simulink model "LLC_FullBridge"  (R2020b)
settings: Solver=VariableStepAuto  StartTime=0.0  StopTime=0.005  MaxStep=1e-4  RelTol=1e-4  EnableMultiTasking=on
PreLoadFcn:
  | Ts_Control=25e-6;
  | Rs_fet=1e8;  % FET snubber resistance (ohms)
  | Cs_fet=inf;  % FET snubber capacitance (ohms)
  | Vf=0.6;        % Diode forward voltage (V)
InitFcn:
  | Ts_Control=25e-6;
libraries: powerlib x24, powerlib_meascontrol x3, pid_lib x1
Description:
  | Copyright 2008-2019 The MathWorks, Inc.
settings Model: SimulationMode=accelerator  Creator=MathWorks  LastModifiedBy=lauramarks2
settings SolverCC: SolverResetMethod=Robust
settings DataIOCC: ReturnWorkspaceOutputs=off
settings OptimizationCC: LifeSpan=inf
settings DebuggingCC: SFUnexpectedBacktrackingDiag=warning  SFNoUnconditionalDefaultTransitionDiag=warning  SFExecutionAtInitializationDiag=none  ArithmeticOperatorsInVariantConditions=warning
settings SFSimCC: SimUseLocalCustomCode=off  CustomCodeUndefinedFunction=UseInterfaceOnly
settings RTWCC: RTWUseLocalCustomCode=off
settings CodeAppCC: StateflowObjectComments=on
settings GRTTargetCC: TargetLangStandard=C89/C90 (ANSI)
settings ConfigComp: CovMetricSettings=dw  CovSaveCumulativeToWorkspaceVar=on  CovSaveSingleToWorkspaceVar=on  CovExternalEMLEnable=off
settings SimscapeCC: SimscapeNormalizeSystem=off  SimscapeNominalValues={1, 'bar'; 1, 'cm^3/s'; 1, 'bar*kg/s'; 1, 'kJ/kg'; 1, 'kW'; }

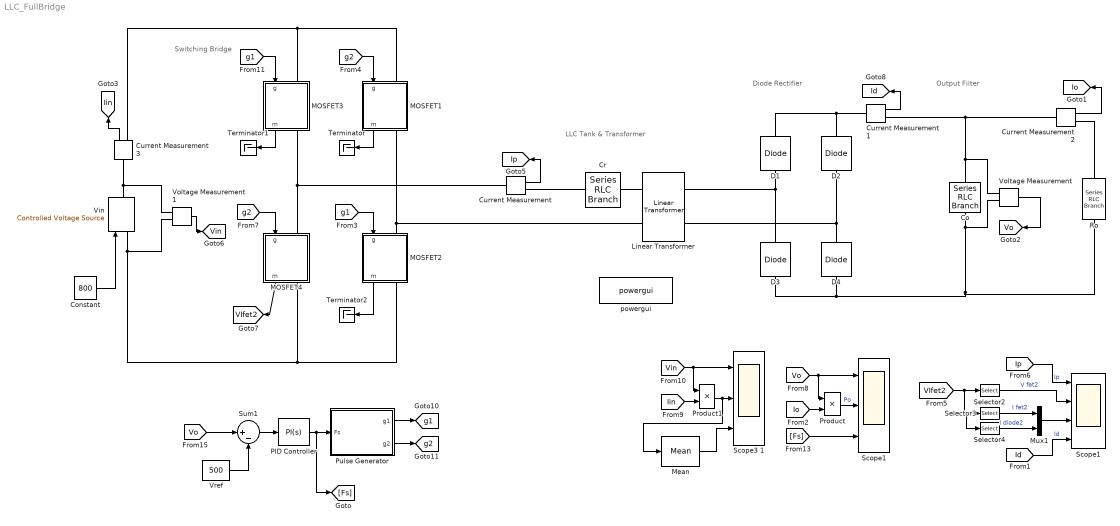
== system LLC_FullBridge ==
  note: LLC Tank & Transformer
  note: Diode
      | Rectifier
  note: Switching
      | Bridge
  note: Output
      | Filter
  Co : powerlib/Elements/Series RLC Branch  LConnTagsString=__new0  RConnTagsString=__new0  BranchType=C  Resistance=1e-4  Inductance=200e-6  SetiL0=off  InitialCurrent=0  Capacitance=100e-6  Setx0=on  InitialVoltage=24  Measurements=None
  Constant : Constant  Value=800  OutDataTypeStr=double
  Cr : powerlib/Elements/Series RLC Branch  LConnTagsString=__new0  RConnTagsString=__new0  BranchType=C  Resistance=1e-4  Inductance=200e-6  SetiL0=off  InitialCurrent=0  Capacitance=1.5e-6  Setx0=off  InitialVoltage=40  Measurements=None
  Current Measurement{,1..3} (4 alike) : powerlib/Measurements/Current Measurement  PhasorSimulation=off  OutputType=Complex  PSBequivalent=0
  D{1..4} (4 alike) : powerlib/Power Electronics/Diode  Ron=1e-3  Lon=0  Vf=0.5  IC=0  UseSnubber=off  Rs=1e6  Cs=inf  Measurements=off
  Linear Transformer : powerlib/Elements/Linear Transformer  UNITS=SI  NominalPower=[ 100e3 85e3 ]  winding1="[8   1e-2  2.02e-6]"  winding2="[6  1e-2  1.16e-6 ]"  ThreeWindings=off  winding3=[3.15e+05 0.7938 0.084225]  RmLm=[1e4 963e-6]  Measurements=None  DataType=on
  MOSFET1 : Subsystem
  MOSFET2 : Subsystem
  MOSFET3 : Subsystem
  MOSFET4 : Subsystem
  Mean : powerlib_meascontrol/Measurements/Mean  Freq=89.2e3  Vinit=0  Ts=0
  Mux1 : Mux  Inputs=2
  PID Controller : pid_lib/PID Controller  Controller=PI  Form=Parallel  TimeDomain=Continuous-time  UseExternalTs=off  SampleTime=-1  IntegratorMethod=Forward Euler  FilterMethod=Forward Euler  ControllerParametersSource=internal  P=1300  I=1e-3  D=0  UseFilter=on  N=100  TunerSelectOption=Transfer Function Based (PID Tuner App)  InitialConditionSource=internal  InitialConditionForIntegrator=89e3  InitialConditionForFilter=0  DifferentiatorICPrevScaledInput=0  ExternalReset=none  TrackingMode=off  Kt=1  LimitOutput=off  SatLimitsSource=internal  UpperSaturationLimit=inf  LowerSaturationLimit=0  LinearizeAsGain=on  AntiWindupMode=none  Kb=1  POutMin=[]  POutMax=[]  IOutMin=[]  IOutMax=[]  DOutMin=[]  DOutMax=[]  NOutMin=[]  NOutMax=[]  SumOutMin=[]  SumOutMax=[]  SaturationOutMin=[]  SaturationOutMax=[]  PParamMin=[]  PParamMax=[]  IParamMin=[]  IParamMax=[]  DParamMin=[]  DParamMax=[]  NParamMin=[]  NParamMax=[]  KbParamMin=[]  KbParamMax=[]  KtParamMin=[]  KtParamMax=[]  KbOutMin=[]  KbOutMax=[]  KtOutMin=[]  KtOutMax=[]  IntegratorOutMin=[]  IntegratorOutMax=[]  FilterOutMin=[]  FilterOutMax=[]  SumI1OutMin=[]  SumI1OutMax=[]  SumI2OutMin=[]  SumI2OutMax=[]  SumI3OutMin=[]  SumI3OutMax=[]  SumI4OutMin=[]  SumI4OutMax=[]  SumDOutMin=[]  SumDOutMax=[]  DifferentiatorOutMin=[]  DifferentiatorOutMax=[]  FilterDiffOutCoefMin=[]  FilterDiffOutCoefMax=[]  ReciprocalOutMin=[]  ReciprocalOutMax=[]  SumDenOutMin=[]  SumDenOutMax=[]  SumNumOutMin=[]  SumNumOutMax=[]  DivideOutMin=[]  DivideOutMax=[]  UdiffTsProdOutMin=[]  UdiffTsProdOutMax=[]  NTsProdOutMin=[]  NTsProdOutMax=[]  UintegralTsProdOutMin=[]  UintegralTsProdOutMax=[]  UngainTsProdOutMin=[]  UngainTsProdOutMax=[]  IntegratorContinuousStateAttributes=''  IntegratorStateMustResolveToSignalObject=off  IntegratorRTWStateStorageClass=Auto  FilterContinuousStateAttributes=''  FilterStateMustResolveToSignalObject=off  FilterRTWStateStorageClass=Auto  ParallelPVariant=InternalParameters  IdealPVariant=Disabled  IVariant=InternalParameters  DVariant=Disabled  IntegratorVariant=Continuous  SatVariant=Disabled  AWVariant=Passthrough  PCopyVariant=Disabled  TRVariant=Disabled  FdbkBlocksVariant=Forward  IdealPFdbkVariant=Disabled  SatFdbkVariant=Disabled  DerivativeFilterVariant=Disabled  NVariant=Disabled  NCopyVariant=Disabled_SignalSpec  FilterICVariant=Disabled  IntegratorICVariant=InternalICs  ExternalResetVariant=Disabled  TRSumVariant=Passthrough  SumFdbkVariant=Disabled  SumVariant=Sum_PI  TsampFilterVariant=InternalTs  TsampNgainVariant=Passthrough  TsampIntegralVariant=Passthrough  ExternalSaturationOutDataTypeStr=Inherit: Same as second input
  Product : Product
  Product1 : Product
  Pulse Generator : Subsystem
  Ro : powerlib/Elements/Series RLC Branch  LConnTagsString=__new0  RConnTagsString=__new0  BranchType=R  Resistance=2.5  Inductance=200e-6  SetiL0=off  InitialCurrent=0  Capacitance=400e-6  Setx0=off  InitialVoltage=0  Measurements=Branch voltage and current
  Scope1 : Scope  NumInputPorts=4
  "Scope1 " : Scope  NumInputPorts=3
  Scope3 1 : Scope  NumInputPorts=3
  Selector2 : Selector  InputPortWidth=3  IndexOptions=Index vector (dialog)  Indices=2  OutputSizes=1
  Selector3 : Selector  InputPortWidth=3  IndexOptions=Index vector (dialog)  Indices=1  OutputSizes=1
  Selector4 : Selector  InputPortWidth=3  IndexOptions=Index vector (dialog)  Indices=3  OutputSizes=1
  Sum1 : Sum  Inputs=|+-  InputSameDT=on  SaturateOnIntegerOverflow=on  OutDataTypeStr=Inherit: Same as first input
  Terminator : Terminator
  Terminator1 : Terminator
  Terminator2 : Terminator
  "Vin " : powerlib/Electrical Sources/Controlled Voltage Source  Initialize=on  Source_Type=AC  Amplitude=0  Phase=0  Frequency=0  Measurements=None
  Voltage Measurement : powerlib/Measurements/Voltage Measurement  PhasorSimulation=off  OutputType=Complex  PSBequivalent=0
  Voltage Measurement1 : powerlib/Measurements/Voltage Measurement  PhasorSimulation=off  OutputType=Complex  PSBequivalent=0
  Vref : Constant  Value=500
  powergui : powerlib/powergui  Priority=1  SimulationMode=Continuous  SampleTime=5e-9  frequency=60  Iterations=50  frequencyindice=0  Pbase=100e6  ErrMax=1e-4  UnitsV=kV  UnitsW=MW  buscounter=0  FunctionMessages=on  echomessages=off  EnableUseOfTLC=off  CurrentSourceSwitches=off  DisableSnubberDevices=off  DisableRonSwitches=off  DisableVfSwitches=off  DisplayEquations=off  AutomaticDiscreteSolvers=off  SolverType=Tustin/Backward Euler (TBE)  Interpol=off  ExternalGateDelay=off  methode=off  Ts=100  x0status=blocks  SPID=on  SwTol=0  HookPort=off  NonlinearTolerance=0  nMaxIteration=15  ContinueOnMaxIteration=off  RestoreLinks=warning  ResistiveCurrentMeasurement=off  Frange=[0:2:500]  Ylog=off  Xlog=on  ShowGrid=off  save=off  variable=ZData  structure=0  ZoomFFT=off  StartTime=0.0  cycles=1  DisplayStyle=1  fundamental=60  FreqAxis=off  MaxFrequency=1000  frequencyindicesteady=1  RmsSteady=1  display=off
  tag scope: Id=global, Iin=global, Io=global, Ip=global, VIfet2=global, Vin=global, Vo=global, g1=global, g2=global
  wires:
  [g1] -> MOSFET2/1(g)
  [g2] -> MOSFET1/1(g)
  Current Measurement/1 -> [Ip]
  Voltage Measurement/1 -> [Vo]
  Current Measurement1/1 -> [Id]
  [Vo] -> Product/1, "Scope1 "/1
  Pulse Generator/1(g1) -> [g1]
  Pulse Generator/2(g2) -> [g2]
  [Fs] -> "Scope1 "/3
  MOSFET1/1(m) -> Terminator/1
  [VIfet2] -> Selector4/1, Selector3/1, Selector2/1
  Mux1/1 -> Scope1/3
  Selector4/1 -> Mux1/2  "I diode2"
  Selector3/1 -> Mux1/1  "I fet2"
  [Id] -> Scope1/4  "Id"
  Selector2/1 -> Scope1/2  "V fet2"
  [Ip] -> Scope1/1  "Ip"
  Current Measurement2/1 -> [Io]
  Product/1 -> "Scope1 "/2  "Po"
  [Io] -> Product/2
  [Vo] -> Sum1/1
  Vref/1 -> Sum1/2
  PID Controller/1 -> [Fs], Pulse Generator/1(Fs)
  Constant/1 -> "Vin "/1
  Sum1/1 -> PID Controller/1
  Current Measurement3/1 -> [Iin]
  [Vin] -> Product1/1, Scope3 1/1
  [Iin] -> Product1/2
  Product1/1 -> Mean/1, Scope3 1/2
  Voltage Measurement1/1 -> [Vin]
  Mean/1 -> Scope3 1/3
  [g2] -> MOSFET4/1(g)
  MOSFET4/1(m) -> [VIfet2]
  [g1] -> MOSFET3/1(g)
  MOSFET3/1(m) -> Terminator1/1
  MOSFET2/1(m) -> Terminator2/1
  connections:
  Co/RConn1 -- Voltage Measurement/LConn2 -- Ro/RConn1 -- D4/LConn1 -- D3/LConn1
  Linear Transformer/RConn1 -- D3/RConn1 -- D1/LConn1
  MOSFET2/LConn1 -- Linear Transformer/LConn2 -- MOSFET1/RConn1
  Linear Transformer/RConn2 -- D4/RConn1 -- D2/LConn1
  MOSFET1/LConn1 -- MOSFET3/LConn1 -- Current Measurement3/RConn1
  "Vin "/LConn1 -- Voltage Measurement1/LConn2 -- MOSFET2/RConn1 -- MOSFET4/RConn1
  Cr/LConn1 -- Current Measurement/RConn1
  Linear Transformer/LConn1 -- Cr/RConn1
  D1/RConn1 -- D2/RConn1 -- Current Measurement1/LConn1
  Voltage Measurement/LConn1 -- Current Measurement2/LConn1 -- Current Measurement1/RConn1 -- Co/LConn1
  Current Measurement2/RConn1 -- Ro/LConn1
  Current Measurement3/LConn1 -- Voltage Measurement1/LConn1 -- "Vin "/RConn1
  MOSFET4/LConn1 -- Current Measurement/LConn1 -- MOSFET3/RConn1

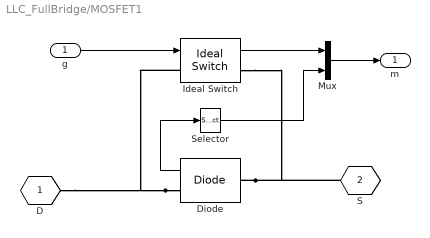
== system LLC_FullBridge/MOSFET1 ==
  g : Inport
  Diode : powerlib/Power Electronics/Diode  Ron=1e-3  Lon=0  Vf=Vf  IC=0  UseSnubber=0  Rs=inf  Cs=0  Measurements=on
  Ideal Switch : powerlib/Power Electronics/Ideal Switch  Ron=1e-3  Lon=0  IC=0  Rs=Rs_fet  Cs=Cs_fet  Measurements=on
  Mux : Mux  Inputs=[2,1]
  Selector : Selector  InputPortWidth=2  IndexOptions=Index vector (dialog)  Indices=1  OutputSizes=1
  D : PMIOPort  Tag=PMCPort  Side=Left
  S : PMIOPort  Tag=PMCPort  Port=2  Side=Right
  m : Outport  VectorParamsAs1DForOutWhenUnconnected=off
  wires:
  Diode/1 -> Selector/1
  g/1 -> Ideal Switch/1
  Ideal Switch/1 -> Mux/1
  Selector/1 -> Mux/2
  Mux/1 -> m/1
  connections:
  Diode/LConn1 -- S/RConn1 -- Ideal Switch/RConn1
  Diode/RConn1 -- D/RConn1 -- Ideal Switch/LConn1

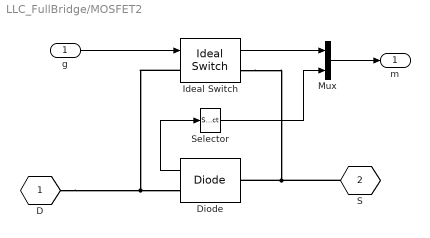
== system LLC_FullBridge/MOSFET2 ==
  g : Inport
  Diode : powerlib/Power Electronics/Diode  Ron=1e-3  Lon=0  Vf=Vf  IC=0  UseSnubber=0  Rs=inf  Cs=0  Measurements=on
  Ideal Switch : powerlib/Power Electronics/Ideal Switch  Ron=1e-3  Lon=0  IC=0  Rs=Rs_fet  Cs=Cs_fet  Measurements=on
  Mux : Mux  Inputs=[2,1]
  Selector : Selector  InputPortWidth=2  IndexOptions=Index vector (dialog)  Indices=1  OutputSizes=1
  D : PMIOPort  Tag=PMCPort  Side=Left
  S : PMIOPort  Tag=PMCPort  Port=2  Side=Right
  m : Outport  VectorParamsAs1DForOutWhenUnconnected=off
  wires:
  Mux/1 -> m/1
  Selector/1 -> Mux/2
  Ideal Switch/1 -> Mux/1
  g/1 -> Ideal Switch/1
  Diode/1 -> Selector/1
  connections:
  Ideal Switch/LConn1 -- D/RConn1 -- Diode/RConn1
  Ideal Switch/RConn1 -- S/RConn1 -- Diode/LConn1

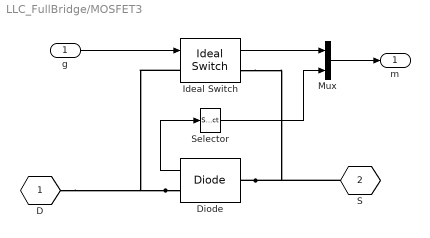
== system LLC_FullBridge/MOSFET3 ==
  g : Inport
  Diode : powerlib/Power Electronics/Diode  Ron=1e-3  Lon=0  Vf=Vf  IC=0  UseSnubber=0  Rs=inf  Cs=0  Measurements=on
  Ideal Switch : powerlib/Power Electronics/Ideal Switch  Ron=1e-3  Lon=0  IC=0  Rs=Rs_fet  Cs=Cs_fet  Measurements=on
  Mux : Mux  Inputs=[2,1]
  Selector : Selector  InputPortWidth=2  IndexOptions=Index vector (dialog)  Indices=1  OutputSizes=1
  D : PMIOPort  Tag=PMCPort  Side=Left
  S : PMIOPort  Tag=PMCPort  Port=2  Side=Right
  m : Outport  VectorParamsAs1DForOutWhenUnconnected=off
  wires:
  Diode/1 -> Selector/1
  g/1 -> Ideal Switch/1
  Ideal Switch/1 -> Mux/1
  Selector/1 -> Mux/2
  Mux/1 -> m/1
  connections:
  Diode/LConn1 -- S/RConn1 -- Ideal Switch/RConn1
  Diode/RConn1 -- D/RConn1 -- Ideal Switch/LConn1

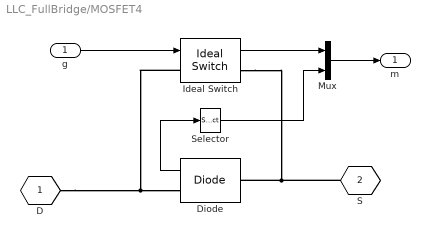
== system LLC_FullBridge/MOSFET4 ==
  g : Inport
  Diode : powerlib/Power Electronics/Diode  Ron=1e-3  Lon=0  Vf=Vf  IC=0  UseSnubber=0  Rs=inf  Cs=0  Measurements=on
  Ideal Switch : powerlib/Power Electronics/Ideal Switch  Ron=1e-3  Lon=0  IC=0  Rs=Rs_fet  Cs=Cs_fet  Measurements=on
  Mux : Mux  Inputs=[2,1]
  Selector : Selector  InputPortWidth=2  IndexOptions=Index vector (dialog)  Indices=1  OutputSizes=1
  D : PMIOPort  Tag=PMCPort  Side=Left
  S : PMIOPort  Tag=PMCPort  Port=2  Side=Right
  m : Outport  VectorParamsAs1DForOutWhenUnconnected=off
  wires:
  Mux/1 -> m/1
  Selector/1 -> Mux/2
  Ideal Switch/1 -> Mux/1
  g/1 -> Ideal Switch/1
  Diode/1 -> Selector/1
  connections:
  Ideal Switch/LConn1 -- D/RConn1 -- Diode/RConn1
  Ideal Switch/RConn1 -- S/RConn1 -- Diode/LConn1

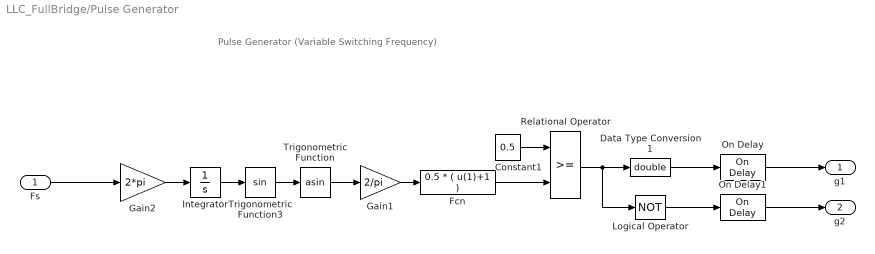
== system LLC_FullBridge/Pulse Generator ==
  note: Pulse Generator
      | (Variable Switching Frequency)
  Fs : Inport
  Constant1 : Constant  Value=0.5
  Data Type Conversion1 : DataTypeConversion  OutDataTypeStr=double
  Fcn : Fcn  Expr=0.5 * ( u(1)+1 )
  Gain1 : Gain  Gain=2/pi  SaturateOnIntegerOverflow=on  OutDataTypeStr=Inherit: Same as input  ParamDataTypeStr=Inherit: Same as input
  Gain2 : Gain  Gain=2*pi  SaturateOnIntegerOverflow=on  OutDataTypeStr=Inherit: Same as input  ParamDataTypeStr=Inherit: Same as input
  Integrator : Integrator
  Logical Operator : Logic  Operator=NOT  AllPortsSameDT=off  OutDataTypeStr=float('double')
  On Delay : powerlib_meascontrol/Logic/On Delay  DelayType=On delay  delay=400e-9  ic=0  Ts=0
  On Delay1 : powerlib_meascontrol/Logic/On Delay  DelayType=On delay  delay=400e-9  ic=0  Ts=0
  Relational Operator : RelationalOperator  OutDataTypeStr=boolean  RndMeth=Nearest
  Trigonometric Function : Trigonometry  Operator=asin
  Trigonometric Function3 : Trigonometry
  g1 : Outport  VectorParamsAs1DForOutWhenUnconnected=off
  g2 : Outport  Port=2  VectorParamsAs1DForOutWhenUnconnected=off
  wires:
  On Delay1/1 -> g2/1
  On Delay/1 -> g1/1
  Fs/1 -> Gain2/1
  Gain2/1 -> Integrator/1
  Data Type Conversion1/1 -> On Delay/1
  Logical Operator/1 -> On Delay1/1
  Fcn/1 -> Relational Operator/2
  Relational Operator/1 -> Logical Operator/1, Data Type Conversion1/1
  Constant1/1 -> Relational Operator/1
  Integrator/1 -> Trigonometric Function3/1
  Trigonometric Function/1 -> Gain1/1
  Gain1/1 -> Fcn/1
  Trigonometric Function3/1 -> Trigonometric Function/1
